simulink model "Controller_C2000"  (R2023a)
settings: Solver=FixedStepDiscrete  StartTime=0.0  StopTime=Inf  RelTol=1e-3  EnableMultiTasking=on
PreLoadFcn:
  | %Pgain = 0.001;           % Controller Proportional Gain
  | %Igain = 0.0001;              % Controller Integral Gain
  | %Dmax = 0.8;                 % Max Duty
  | %FPWM1 = 100e3;              % PWM1 Frequency
  | 
  | % PWM1 100Khz switching Frequency
  | %TBPRD1 = 600;
  | % hardwareParameters;
model workspace (MAT data in the model file):
  op : simscape.op.OperatingPoint (value not decoded)
libraries: c2806xlib x5, svdutilitieslib x4, c280xlib x2, c2000lib x1
settings Model: DataDictionary=ControlParams.sldd  EnableAccessToBaseWorkspace=off  SimulationMode=external  ExtModeTrigDuration=8  ExtModeTrigLevel=0.500000  ExtModeArchiveMode=auto  ExtModeArchiveFileName=output.mat  ExtModeArchiveDirName=C:\VersionControl\Git\TIC2000_DCDC_LED\Data\Recording  Creator=vivekr  LastModifiedBy=ppatel
settings SolverCC: AlgebraicLoopSolver=TrustRegion
settings DataIOCC: Decimation=5  LimitDataPoints=on  MaxDataPoints=15000  SaveFinalState=on  SaveOutput=off  SaveTime=off  ReturnWorkspaceOutputs=off
settings OptimizationCC: DefaultUnderspecifiedDataType=single  UseSpecifiedMinMax=on  EnhancedBackFolding=on  StrengthReduction=on  PassReuseOutputArgsAs=Individual arguments  NoFixptDivByZeroProtection=on  EfficientFloat2IntCast=on  LifeSpan=1  MaxStackSize=1024  DenormalBehavior=FlushToZero  EfficientTunableParamExpr=on
settings DebuggingCC: SolverPrmCheckMsg=warning  ParameterPrecisionLossMsg=none  UnconnectedInputMsg=warning  UnconnectedOutputMsg=warning  UnconnectedLineMsg=warning  AllowSymbolicDim=off  PregeneratedLibrarySubsystemCodeDiagnostic=none  SFUnexpectedBacktrackingDiag=warning  SFNoUnconditionalDefaultTransitionDiag=warning  SFExecutionAtInitializationDiag=none  ArithmeticOperatorsInVariantConditions=warning
settings HardwareCC: ProdBitPerChar=16  ProdBitPerInt=16  ProdBitPerPointer=32  ProdBitPerSizeT=32  ProdBitPerPtrDiffT=32  ProdLargestAtomicInteger=Integer  ProdLargestAtomicFloat=None  ProdWordSize=16  ProdLongLongMode=on  ProdHWDeviceType=Texas Instruments->C2000
settings ModelReferenceCC: EnableRefExpFcnMdlSchedulingChecks=on  ModelReferenceNumInstancesAllowed=Single  PropagateSignalLabelsOutOfModel=off
settings SFSimCC: SimUseLocalCustomCode=off  MATLABDynamicMemAlloc=off  CustomCodeUndefinedFunction=UseInterfaceOnly
settings RTWCC: Description=Embedded Coder  SystemTargetFile=ert.tlc  HardwareBoard=TI Piccolo F2806x  TemplateMakefile=ert_default_tmf  RTWUseLocalCustomCode=off  Toolchain=Texas Instruments Code Composer Studio (C2000)  BuildConfiguration=Faster Runs  IncludeHyperlinkInReport=on  CodeProfilingSaveOptions=AllData  DLArmComputeVersion=19.05
settings CodeAppCC: IgnoreCustomStorageClasses=off  StateflowObjectComments=on
settings ERTTargetCC: CodeReplacementLibrary=TI C28x  MultiwordLength=2048  IncludeMdlTerminateFcn=off  CombineSignalStateStructs=on  SupportNonFinite=off  SupportComplex=off  ExtMode=on  ExtModeTransport=3  ExtModeStaticAllocSize=2000  ExtModeMexArgs='127.0.0.1' 0 17725  ERTFilePackagingFormat=Compact
settings ConfigComp: CovMetricSettings=dw  CovSaveCumulativeToWorkspaceVar=on  CovSaveSingleToWorkspaceVar=on  CovExternalEMLEnable=off  CovSFcnEnable=off
settings SimscapeCC: SimscapeNormalizeSystem=off  SimscapeLogName=simlog_OP  SimscapeLogLimitData=off  SimscapeOperatingPoint=op

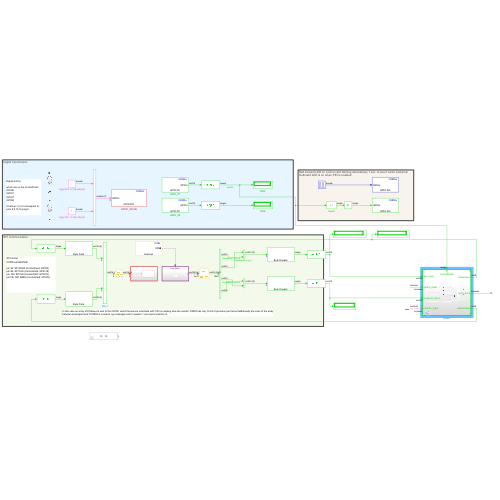
[thumbnail: Simulink's stored preview of the top-level diagram]
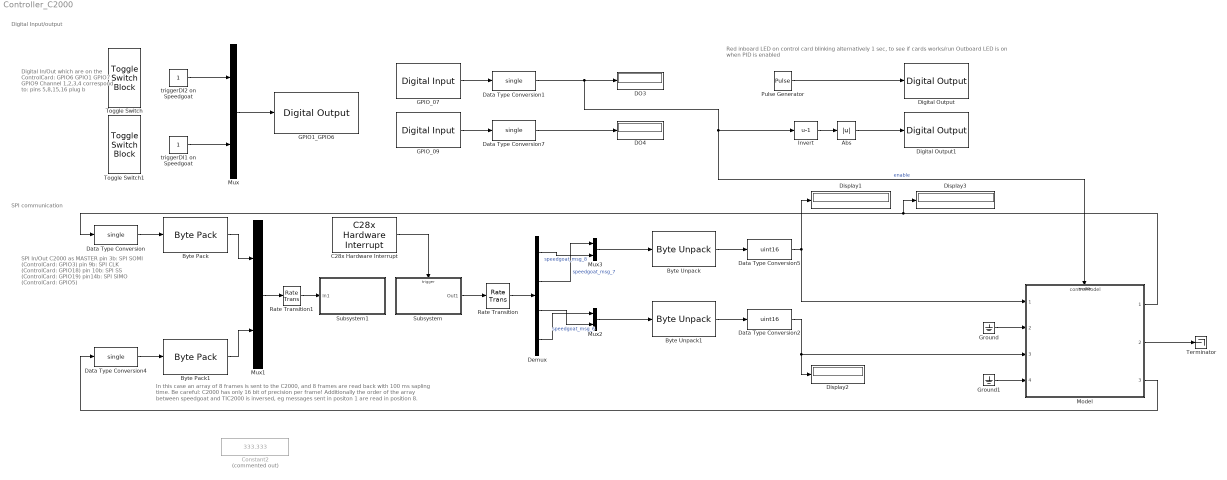
== system Controller_C2000 ==
  note: SPI communication
  note: Digital Input/output
  note: In this case an array of 8 frames is sent to the C2000, and 8 frames are read back with 100 ms sapling time. Be careful: C2000 has only 16 bit of precision per frame! Additionally the order of the array
      | between speedgoat and TIC2000 is inversed, eg messages sent in positon 1 are read in position 8.
  note: Red inboard LED on control card blinking alternatively 1 sec, to see if cards works/run
      | Outboard LED is on when PID is enabled
  note: Digital In/Out
      |
      | which are on the ControlCard:
      | GPIO6
      | GPIO1
      | GPIO7
      | GPIO9
      |
      | Channel 1,2,3,4 correspond to:
      | pins 5,8,15,16 plug b
  note: SPI In/Out
      | C2000 as MASTER
      |
      | pin 3b: SPI SOMI (ControlCard: GPIO3)
      | pin 9b: SPI CLK (ControlCard: GPIO18)
      | pin 10b: SPI SS (ControlCard: GPIO19)
      | pin14b: SPI SIMO (ControlCard: GPIO5)
  Abs : Abs  SaturateOnIntegerOverflow=off
  Byte Pack : svdutilitieslib/Byte Pack  maskPackedDataType=uint16  datatypes={'single'}  byteAlign=2  blockPlatform=tic2000
  Byte Pack1 : svdutilitieslib/Byte Pack  maskPackedDataType=uint16  datatypes={'single'}  byteAlign=2  blockPlatform=tic2000
  Byte Unpack : svdutilitieslib/Byte Unpack  dimensions={[1]}  datatypes={'single'}  byteAlign=2  blockPlatform=tic2000
  Byte Unpack1 : svdutilitieslib/Byte Unpack  dimensions={[1]}  datatypes={'single'}  byteAlign=2  blockPlatform=tic2000
  C28x Hardware Interrupt : c2000lib/Scheduling/C28x Hardware Interrupt  irqnumbers=6  pienumbers=1  irqpriorities=30  irqpreempts=1  showinput=off  dspchiptype=C280X
  Constant2 : Constant  Commented=on  Value=333.333  SampleTime=-1
  DO3 : Display
  DO4 : Display
  Data Type Conversion{,1,4,7} (4 alike) : DataTypeConversion  OutDataTypeStr=single  SaturateOnIntegerOverflow=off  RndMeth=Floor
  Data Type Conversion2 : DataTypeConversion  OutDataTypeStr=uint16  SaturateOnIntegerOverflow=off  RndMeth=Floor
  Data Type Conversion5 : DataTypeConversion  OutDataTypeStr=uint16  SaturateOnIntegerOverflow=off  RndMeth=Floor
  Demux : Demux
  Digital Output : c2806xlib/Digital Output  GPIO_Number=GPIO24~GPIO31  GPIO_Bit0=off  GPIO_BIT0_Toggle=off  GPIO_Bit1=off  GPIO_BIT1_Toggle=off  GPIO_Bit2=off  GPIO_BIT2_Toggle=off  GPIO_Bit3=off  GPIO_BIT3_Toggle=off  GPIO_Bit4=off  GPIO_BIT4_Toggle=off  GPIO_Bit5=off  GPIO_BIT5_Toggle=off  GPIO_Bit6=off  GPIO_BIT6_Toggle=off  GPIO_Bit7=on  GPIO_BIT7_Toggle=off
  Digital Output1 : c2806xlib/Digital Output  GPIO_Number=GPIO32~GPIO39  GPIO_Bit0=off  GPIO_BIT0_Toggle=off  GPIO_Bit1=off  GPIO_BIT1_Toggle=off  GPIO_Bit2=on  GPIO_BIT2_Toggle=off  GPIO_Bit3=off  GPIO_BIT3_Toggle=off  GPIO_Bit4=off  GPIO_BIT4_Toggle=off  GPIO_Bit5=off  GPIO_BIT5_Toggle=off  GPIO_Bit6=off  GPIO_BIT6_Toggle=off  GPIO_Bit7=off  GPIO_BIT7_Toggle=off
  Display1 : Display
  Display2 : Display
  Display3 : Display
  GPIO1_GPIO6 : c2806xlib/Digital Output  GPIO_Number=GPIO0~GPIO7  GPIO_Bit0=off  GPIO_BIT0_Toggle=off  GPIO_Bit1=on  GPIO_BIT1_Toggle=off  GPIO_Bit2=off  GPIO_BIT2_Toggle=off  GPIO_Bit3=off  GPIO_BIT3_Toggle=off  GPIO_Bit4=off  GPIO_BIT4_Toggle=off  GPIO_Bit5=off  GPIO_BIT5_Toggle=off  GPIO_Bit6=on  GPIO_BIT6_Toggle=off  GPIO_Bit7=off  GPIO_BIT7_Toggle=off
  GPIO_07 : c2806xlib/Digital Input  GPIO_Number=GPIO0~GPIO7  GPIO_Bit0=off  GPIO_Bit1=off  GPIO_Bit2=off  GPIO_Bit3=off  GPIO_Bit4=off  GPIO_Bit5=off  GPIO_Bit6=off  GPIO_Bit7=on  sampleTime=1e-2  dataType=auto  GPIO_Bit0_Qualification=Sync to SYSCLKOUT  GPIO_Bit1_Qualification=Sync to SYSCLKOUT  GPIO_Bit2_Qualification=Sync to SYSCLKOUT  GPIO_Bit3_Qualification=Sync to SYSCLKOUT  GPIO_Bit4_Qualification=Sync to SYSCLKOUT  GPIO_Bit5_Qualification=Sync to SYSCLKOUT  GPIO_Bit6_Qualification=Sync to SYSCLKOUT  GPIO_Bit7_Qualification=Sync to SYSCLKOUT  Qualification_Period=-1
  GPIO_09 : c2806xlib/Digital Input  GPIO_Number=GPIO8~GPIO15  GPIO_Bit0=off  GPIO_Bit1=on  GPIO_Bit2=off  GPIO_Bit3=off  GPIO_Bit4=off  GPIO_Bit5=off  GPIO_Bit6=off  GPIO_Bit7=off  sampleTime=1e-2  dataType=auto  GPIO_Bit0_Qualification=Sync to SYSCLKOUT  GPIO_Bit1_Qualification=Sync to SYSCLKOUT  GPIO_Bit2_Qualification=Sync to SYSCLKOUT  GPIO_Bit3_Qualification=Sync to SYSCLKOUT  GPIO_Bit4_Qualification=Sync to SYSCLKOUT  GPIO_Bit5_Qualification=Sync to SYSCLKOUT  GPIO_Bit6_Qualification=Sync to SYSCLKOUT  GPIO_Bit7_Qualification=Sync to SYSCLKOUT  Qualification_Period=-1
  Ground : Ground
  Ground1 : Ground
  Invert : Bias  Bias=-1  SaturateOnIntegerOverflow=off
  Model : ModelReference  ModelNameDialog=controlModel.slx  SimulationMode=Normal  ModelReferenceVersion=8.10  EnablePortName=Enable  EnablePortStatesWhenEnabling=reset
  Mux{,1..3} (4 alike) : Mux  Inputs=2
  Pulse Generator : DiscretePulseGenerator  PulseType=Time based  PulseWidth=50
  Rate Transition : RateTransition  Deterministic=off
  Rate Transition1 : RateTransition  Deterministic=off
  Subsystem : Subsystem
  Subsystem1 : Subsystem  TreatAsAtomicUnit=on  SystemSampleTime=0.001
  Terminator : Terminator
  Toggle Switch : ToggleSwitchBlock  LabelPosition=Hide
      settings: Values={{'Off', 'On'}, [0 1]}
  Toggle Switch1 : ToggleSwitchBlock  LabelPosition=Hide
      settings: Values={{'Off', 'On'}, [0 1]}
  triggerDI1 on Speedgoat : Constant
  triggerDI2 on Speedgoat : Constant
  wires:
  Pulse Generator/1 -> Digital Output/1
  Data Type Conversion1/1 -> DO3/1, Model/Enable, Invert/1  "enable"
  Mux/1 -> GPIO1_GPIO6/1
  triggerDI2 on Speedgoat/1 -> Mux/1
  triggerDI1 on Speedgoat/1 -> Mux/2
  GPIO_07/1 -> Data Type Conversion1/1
  GPIO_09/1 -> Data Type Conversion7/1
  Data Type Conversion7/1 -> DO4/1
  Demux/1 -> Mux3/2  "speedgoat_msg_8"
  Demux/2 -> Mux3/1  "speedgoat_msg_7"
  C28x Hardware Interrupt/1 -> Subsystem/Trigger
  Mux3/1 -> Byte Unpack/1
  Byte Unpack/1 -> Data Type Conversion5/1
  Data Type Conversion5/1 -> Model/1, Display1/1
  Byte Unpack1/1 -> Data Type Conversion2/1
  Mux2/1 -> Byte Unpack1/1
  Demux/3 -> Mux2/2  "speedgoat_msg_6"
  Demux/4 -> Mux2/1
  Subsystem/1(Out1) -> Rate Transition/1
  Mux1/1 -> Rate Transition1/1
  Model/3 -> Data Type Conversion4/1
  Rate Transition/1 -> Demux/1
  Data Type Conversion/1 -> Byte Pack/1
  Byte Pack/1 -> Mux1/1
  Data Type Conversion4/1 -> Byte Pack1/1
  Byte Pack1/1 -> Mux1/2
  Model/1 -> Display3/1, Data Type Conversion/1
  Data Type Conversion2/1 -> Model/3, Display2/1
  Abs/1 -> Digital Output1/1
  Invert/1 -> Abs/1
  Ground/1 -> Model/2
  Ground1/1 -> Model/4
  Model/2 -> Terminator/1
  Rate Transition1/1 -> Subsystem1/1(In1)

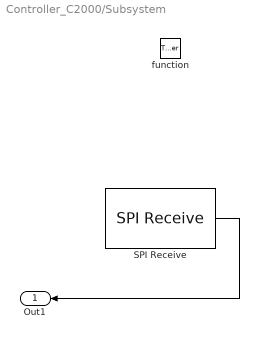
== system Controller_C2000/Subsystem ==
  function : TriggerPort  TriggerType=function-call  VariantControl=Variant
  SPI Receive : c280xlib/SPI Receive  SPISelect=SPI_A  ClockPolarity=Rising_edge  ClockPhase=No_delay  SPIModule=uint32(0)  Mode=Master  BusSpeed=uint32(1000000)  FirstBitToTransfer=Most significant bit (MSB)  ClockMode=0  BlockFunction=Read  EnableRegisterAddress=on  RegisterAddress=0  OutputDataType=uint16  OutputDataLength=4  BlockingMode=on  SampleTime=-1  DataBits=16  UseCustomSSPin=Provided by the SPI peripheral  ActiveLowSSPin=Active low  Pin=0
  Out1 : Outport
  wires:
  SPI Receive/1 -> Out1/1

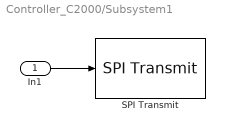
== system Controller_C2000/Subsystem1 ==
  In1 : Inport
  SPI Transmit : c280xlib/SPI Transmit  SPISelect=SPI_A  ClockPolarity=Rising_edge  ClockPhase=No_delay  SPIModule=uint32(0)  Mode=Master  BusSpeed=uint32(1000000)  FirstBitToTransfer=Most significant bit (MSB)  ClockMode=0  BlockFunction=Write  EnableRegisterAddress=on  RegisterAddress=0  OutputDataType=int8  OutputDataLength=1  BlockingMode=on  DataBits=16  UseCustomSSPin=Provided by the SPI peripheral  ActiveLowSSPin=Active low  Pin=0
  wires:
  In1/1 -> SPI Transmit/1
